simulink model "sim_model_withparasitic_rlload_before"  (R2016a)
settings: Solver=ode4  StartTime=0.0  StopTime=Tfinal  FixedStep=Ts  RelTol=1e-3
values from neighbouring files (symbols this model uses):
  Cdc1 = 5e-6    (= 5e-06)    [sim_parameters.m]    (also in sim_parameters_parallel.m; sim_parameters_rl_load.m)
  delta = acos(Ef/Vt)    [sim_parameters.m]    (also in sim_parameters_parallel.m; sim_parameters_rl_load.m = 0)
  deltad = delta*180/pi    [sim_parameters.m]    (also in sim_parameters_parallel.m; sim_parameters_rl_load.m = 0)
  ESL = 19e-15    (= 1.9e-14)    [sim_parameters.m]    (also in sim_parameters_parallel.m; sim_parameters_rl_load.m = 1e-15)
  ESR = 21.1e-15    (= 2.11e-14)    [sim_parameters.m]    (also in sim_parameters_parallel.m; sim_parameters_rl_load.m = 1e-15)
  LABBot = 10.20e-9    (= 1.02e-08)    [impedance_inductancemodel.m]    (also in sim_parameters_rl_load.m = 1.02e-14)
  LABot = 20.25e-9    (= 2.025e-08)    [impedance_inductancemodel.m]    (also in sim_parameters_rl_load.m = 2.025e-14)
  LABTop = 18.30e-9    (= 1.83e-08)    [impedance_inductancemodel.m]    (also in sim_parameters_rl_load.m = 1.83e-14)
  LATop = 03.40e-9    (= 3.4e-09)    [impedance_inductancemodel.m]    (also in sim_parameters_rl_load.m = 3.4e-15)
  LBBot = 20.38e-9    (= 2.038e-08)    [impedance_inductancemodel.m]    (also in sim_parameters_rl_load.m = 2.038e-14)
  LBCBot = 11.14e-9    (= 1.114e-08)    [impedance_inductancemodel.m]    (also in sim_parameters_rl_load.m = 1.114e-14)
  LBTop = 03.38e-9    (= 3.38e-09)    [impedance_inductancemodel.m]    (also in sim_parameters_rl_load.m = 3.38e-15)
  LCBot = 20.94e-9    (= 2.094e-08)    [impedance_inductancemodel.m]    (also in sim_parameters_rl_load.m = 2.094e-14)
  LCTop = 03.41e-9    (= 3.41e-09)    [impedance_inductancemodel.m]    (also in sim_parameters_rl_load.m = 3.41e-15)
  Lin = 1e-15    [sim_parameters.m]    (also in sim_parameters_parallel.m; sim_parameters_rl_load.m = 1e-06)
  Lload = Xload/(2*pi*fout)    [sim_parameters_rl_load.m]
  ma = Vt*sqrt(3)/(Vdcm*0.612)    [sim_parameters.m]    (also in sim_parameters_parallel.m; sim_parameters_rl_load.m = 0.9)
  maxlim = 340    [sim_parameters.m]    (also in sim_parameters_parallel.m; sim_parameters_rl_load.m)
  minlim = 200    [sim_parameters.m]    (also in sim_parameters_parallel.m; sim_parameters_rl_load.m)
  phase = [0 90 0 90]    [sim_parameters.m]    (also in sim_parameters_parallel.m = [0 0]; sim_parameters_rl_load.m = [0 0])
  RABBot = 10.20e-15    (= 1.02e-14)    [sim_parameters_rl_load.m]
  RABot = 20.25e-15    (= 2.025e-14)    [sim_parameters_rl_load.m]
  RABTop = 18.30e-15    (= 1.83e-14)    [sim_parameters_rl_load.m]
  RATop = 03.40e-15    (= 3.4e-15)    [sim_parameters_rl_load.m]
  RBBot = 20.38e-15    (= 2.038e-14)    [sim_parameters_rl_load.m]
  RBCBot = 11.14e-15    (= 1.114e-14)    [sim_parameters_rl_load.m]
  RBCTop = 21.84e-15    (= 2.184e-14)    [sim_parameters_rl_load.m]
  RBTop = 03.38e-15    (= 3.38e-15)    [sim_parameters_rl_load.m]
  RCBot = 20.94e-15    (= 2.094e-14)    [sim_parameters_rl_load.m]
  RCTop = 03.41e-15    (= 3.41e-15)    [sim_parameters_rl_load.m]
  Rin = 70    [sim_parameters.m]    (also in sim_parameters_parallel.m = 50; sim_parameters_rl_load.m = 200)
  Ripth = 0.3    [sim_parameters.m]    (also in sim_parameters_parallel.m; sim_parameters_rl_load.m = 0.03)
  Rload = Zload*pf    [sim_parameters_rl_load.m]
  Ts = 1e-6    (= 1e-06)    [sim_parameters.m]    (also in sim_parameters_parallel.m = 1e-07; sim_parameters_rl_load.m = 1e-08)
  Vin = Vdc + Rin*(Pout/Vdc)    (= 1751.48148148)    [sim_parameters_rl_load.m]
  wout = 2*pi*fout    (= 314.159265359)    [sim_parameters.m]    (also in sim_parameters_parallel.m; sim_parameters_rl_load.m)
libraries: powerlib x38, powerlib_meascontrol x9, simulink x2
settings Model: SimulationMode=accelerator  Creator=ugurm  LastModifiedBy=mesutto
settings DataIOCC: LimitDataPoints=on  SaveFormat=Array
settings OptimizationCC: EfficientMapNaN2IntZero=off
settings DebuggingCC: UnderspecifiedInitializationDetection=Classic  MergeDetectMultiDrivingBlocksExec=none  SolverPrmCheckMsg=warning  StateNameClashWarn=warning
settings HardwareCC: ProdBitPerPointer=32  ProdLargestAtomicFloat=None  ProdIntDivRoundTo=Undefined  ProdEndianess=Unspecified  ProdWordSize=32  ProdHWDeviceType=32-bit Generic  TargetBitPerPointer=64  TargetLongLongMode=on  TargetIntDivRoundTo=Zero  TargetEndianess=LittleEndian  TargetWordSize=64  TargetHWDeviceType=MATLAB Host  ProdEqTarget=off
settings ModelReferenceCC: PropagateSignalLabelsOutOfModel=off
settings CodeAppCC: MaxIdLength=128
settings GRTTargetCC: GeneratePreprocessorConditionals=Use local settings  CombineOutputUpdateFcns=off  GRTInterface=on
settings ConfigComp: CovModelRefEnable=Off

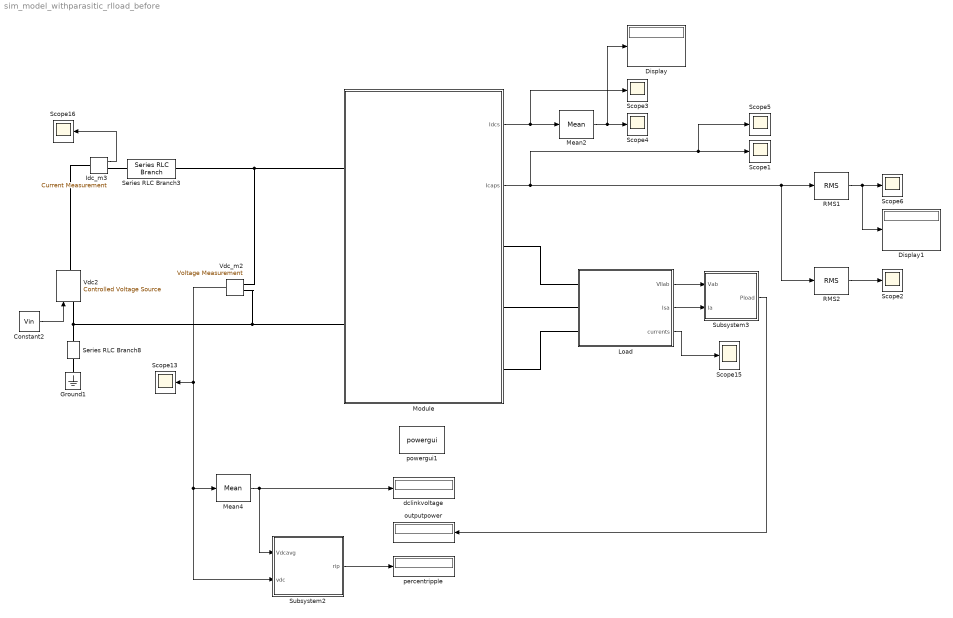
== system sim_model_withparasitic_rlload_before ==
  Constant2 : Constant  Value=Vin
  Display : Display
  Display1 : Display
  Ground1 : powerlib/Elements/Ground  LConnTagsString=a
  Idc_m3 : powerlib/Measurements/Current Measurement  PhasorSimulation=off  OutputType=Complex  PSBequivalent=0
  Load : Subsystem
  Mean2 : powerlib_meascontrol/Measurements/Mean  Freq=fout  Vinit=0  Ts=0
  Mean4 : powerlib_meascontrol/Measurements/Mean  Freq=fout  Vinit=0  Ts=0
  Module : Subsystem
  RMS1 : powerlib_meascontrol/Measurements/RMS  TrueRMS=on  Freq=fout  RMSInit=0  Ts=0
  RMS2 : powerlib_meascontrol/Measurements/RMS  TrueRMS=on  Freq=fsw  RMSInit=0  Ts=0
  Scope{1..6,13,15..16} (9 alike) : Scope
  Series RLC Branch3 : powerlib/Elements/Series RLC Branch  LConnTagsString=__new0  RConnTagsString=__new0  BranchType=R  Resistance=Rin  Inductance=Lin  SetiL0=off  InitialCurrent=0  Capacitance=1e-6  Setx0=off  InitialVoltage=0  Measurements=None
  Series RLC Branch8 : powerlib/Elements/Series RLC Branch  LConnTagsString=__new0  RConnTagsString=__new0  BranchType=R  Resistance=1e12  Inductance=Lload  SetiL0=off  InitialCurrent=0  Capacitance=1e-6  Setx0=off  InitialVoltage=0  Measurements=None
  Subsystem2 : Subsystem
  Subsystem3 : Subsystem
  Vdc2 : powerlib/Electrical Sources/Controlled Voltage Source  Initialize=off  Source_Type=DC  Amplitude=200  Phase=0  Frequency=0  Measurements=None
  Vdc_m2 : powerlib/Measurements/Voltage Measurement  PhasorSimulation=off  OutputType=Complex  PSBequivalent=0
  dclinkvoltage : Display
  outputpower : Display
  percentripple : Display
  powergui1 : powerlib/powergui  Priority=1  SimulationMode=Discrete  SolverType=Tustin  SampleTime=Ts  frequency=60  SPID=off  DisableSnubberDevices=off  DisableRonSwitches=off  DisableVfSwitches=off  SwTol=0  DisplayEquations=off  Interpol=off  ExternalGateDelay=off  methode=off  Ts=0  FunctionMessages=off  echomessages=off  HookPort=off  EnableUseOfTLC=off  x0status=blocks  frequencyindice=0  Pbase=100e6  ErrMax=1e-4  Iterations=50  UnitsV=kV  UnitsW=MW  buscounter=0  RestoreLinks=warning  ResistiveCurrentMeasurement=off  Frange=[0:2:500]  Ylog=off  Xlog=on  ShowGrid=off  save=off  variable=ZData  structure=vdc  ZoomFFT=off  StartTime=0.35  cycles=5  DisplayStyle=4  fundamental=50  FreqAxis=off  MaxFrequency=50000  frequencyindicesteady=1  RmsSteady=1  display=off
  wires:
  Constant2/1 -> Vdc2/1
  Mean4/1 -> Subsystem2/1(Vdcavg), dclinkvoltage/1
  Vdc_m2/1 -> Scope13/1, Subsystem2/2(vdc), Mean4/1
  Idc_m3/1 -> Scope16/1
  Subsystem3/1(Pload) -> outputpower/1
  Load/1(Vllab) -> Subsystem3/1(Vab)
  Load/2(Isa) -> Subsystem3/2(Ia)
  Load/3(currents) -> Scope15/1
  Module/1(Idcs) -> Mean2/1, Scope3/1
  Mean2/1 -> Display/1, Scope4/1
  Module/2(Icaps) -> RMS2/1, RMS1/1, Scope1/1, Scope5/1
  RMS1/1 -> Display1/1, Scope6/1
  Subsystem2/1(rip) -> percentripple/1
  RMS2/1 -> Scope2/1
  connections:
  Series RLC Branch8/RConn1 -- Ground1/LConn1
  Idc_m3/RConn1 -- Series RLC Branch3/LConn1
  Idc_m3/LConn1 -- Vdc2/RConn1
  Vdc_m2/LConn2 -- Module/LConn2 -- Series RLC Branch8/LConn1 -- Vdc2/LConn1
  Vdc_m2/LConn1 -- Series RLC Branch3/RConn1 -- Module/LConn1
  Load/LConn1 -- Module/RConn1
  Load/LConn2 -- Module/RConn2
  Load/LConn3 -- Module/RConn3

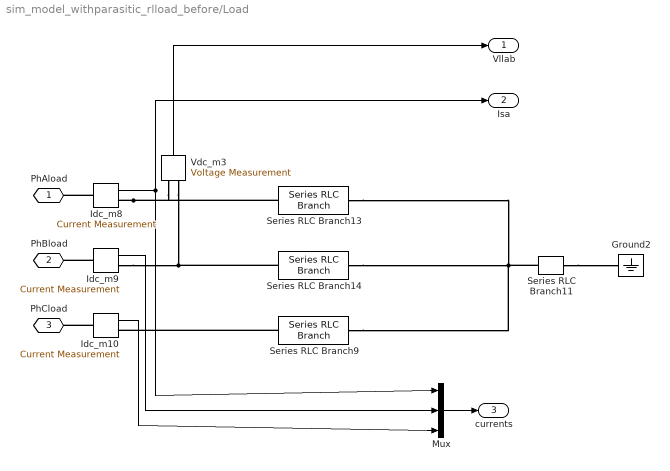
== system sim_model_withparasitic_rlload_before/Load ==
  Ground2 : powerlib/Elements/Ground  LConnTagsString=a
  Idc_m10 : powerlib/Measurements/Current Measurement  PhasorSimulation=off  OutputType=Complex  PSBequivalent=0
  Idc_m8 : powerlib/Measurements/Current Measurement  PhasorSimulation=off  OutputType=Complex  PSBequivalent=0
  Idc_m9 : powerlib/Measurements/Current Measurement  PhasorSimulation=off  OutputType=Complex  PSBequivalent=0
  Mux : Mux  Inputs=3
  Series RLC Branch11 : powerlib/Elements/Series RLC Branch  LConnTagsString=__new0  RConnTagsString=__new0  BranchType=R  Resistance=1e12  Inductance=Lload  SetiL0=off  InitialCurrent=0  Capacitance=1e-6  Setx0=off  InitialVoltage=0  Measurements=None
  Series RLC Branch13 : powerlib/Elements/Series RLC Branch  LConnTagsString=__new0  RConnTagsString=__new0  BranchType=RL  Resistance=Rload  Inductance=Lload  SetiL0=off  InitialCurrent=0  Capacitance=1e-6  Setx0=off  InitialVoltage=0  Measurements=None
  Series RLC Branch14 : powerlib/Elements/Series RLC Branch  LConnTagsString=__new0  RConnTagsString=__new0  BranchType=RL  Resistance=Rload  Inductance=Lload  SetiL0=off  InitialCurrent=0  Capacitance=1e-6  Setx0=off  InitialVoltage=0  Measurements=None
  Series RLC Branch9 : powerlib/Elements/Series RLC Branch  LConnTagsString=__new0  RConnTagsString=__new0  BranchType=RL  Resistance=Rload  Inductance=Lload  SetiL0=off  InitialCurrent=0  Capacitance=1e-6  Setx0=off  InitialVoltage=0  Measurements=None
  Vdc_m3 : powerlib/Measurements/Voltage Measurement  PhasorSimulation=off  OutputType=Complex  PSBequivalent=0
  PhAload : PMIOPort  Port=1  Side=Left
  PhBload : PMIOPort  Port=2  Side=Left
  PhCload : PMIOPort  Port=3  Side=Left
  Vllab : Outport
  Isa : Outport  Port=2
  currents : Outport  Port=3
  wires:
  Vdc_m3/1 -> Vllab/1
  Idc_m9/1 -> Mux/2
  Idc_m10/1 -> Mux/3
  Idc_m8/1 -> Mux/1, Isa/1
  Mux/1 -> currents/1
  connections:
  Idc_m10/LConn1 -- PhCload/RConn1
  Idc_m9/LConn1 -- PhBload/RConn1
  Idc_m8/LConn1 -- PhAload/RConn1
  Series RLC Branch9/LConn1 -- Idc_m10/RConn1
  Vdc_m3/LConn2 -- Idc_m9/RConn1 -- Series RLC Branch14/LConn1
  Series RLC Branch13/RConn1 -- Series RLC Branch9/RConn1 -- Series RLC Branch11/LConn1 -- Series RLC Branch14/RConn1
  Idc_m8/RConn1 -- Vdc_m3/LConn1 -- Series RLC Branch13/LConn1
  Series RLC Branch11/RConn1 -- Ground2/LConn1

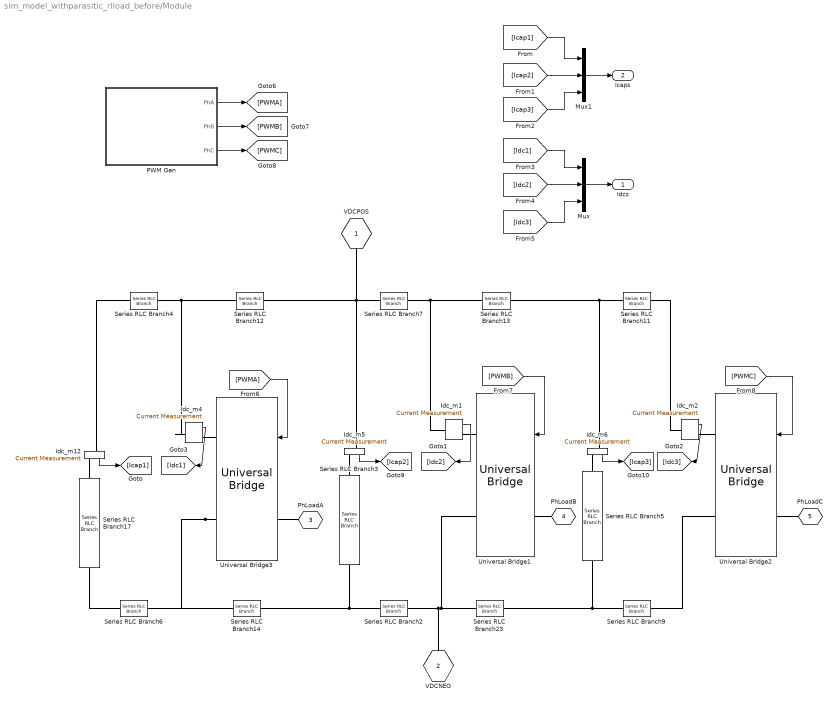
== system sim_model_withparasitic_rlload_before/Module ==
  Idc_m{1..2,4..6,12} (6 alike) : powerlib/Measurements/Current Measurement  PhasorSimulation=off  OutputType=Complex  PSBequivalent=0
  Mux : Mux  Inputs=3
  Mux1 : Mux  Inputs=3
  PWM Gen : Subsystem
  Series RLC Branch11 : powerlib/Elements/Series RLC Branch  LConnTagsString=__new0  RConnTagsString=__new0  BranchType=RL  Resistance=RCTop  Inductance=LCTop  SetiL0=off  InitialCurrent=0  Capacitance=1e-6  Setx0=off  InitialVoltage=0  Measurements=None
  Series RLC Branch12 : powerlib/Elements/Series RLC Branch  LConnTagsString=__new0  RConnTagsString=__new0  BranchType=RL  Resistance=RABTop  Inductance=LABTop  SetiL0=off  InitialCurrent=0  Capacitance=1e-6  Setx0=off  InitialVoltage=0  Measurements=None
  Series RLC Branch13 : powerlib/Elements/Series RLC Branch  LConnTagsString=__new0  RConnTagsString=__new0  BranchType=RL  Resistance=RBCTop  Inductance=RBCTop  SetiL0=off  InitialCurrent=0  Capacitance=1e-6  Setx0=off  InitialVoltage=0  Measurements=None
  Series RLC Branch14 : powerlib/Elements/Series RLC Branch  LConnTagsString=__new0  RConnTagsString=__new0  BranchType=RL  Resistance=RABBot  Inductance=LABBot  SetiL0=off  InitialCurrent=0  Capacitance=1e-6  Setx0=off  InitialVoltage=0  Measurements=None
  Series RLC Branch17 : powerlib/Elements/Series RLC Branch  LConnTagsString=__new0  RConnTagsString=__new0  BranchType=RLC  Resistance=ESR  Inductance=ESL  SetiL0=off  InitialCurrent=0  Capacitance=Cdc1  Setx0=off  InitialVoltage=0  Measurements=None
  Series RLC Branch2 : powerlib/Elements/Series RLC Branch  LConnTagsString=__new0  RConnTagsString=__new0  BranchType=RL  Resistance=RBBot  Inductance=LBBot  SetiL0=off  InitialCurrent=0  Capacitance=1e-6  Setx0=off  InitialVoltage=0  Measurements=None
  Series RLC Branch23 : powerlib/Elements/Series RLC Branch  LConnTagsString=__new0  RConnTagsString=__new0  BranchType=RL  Resistance=RBCBot  Inductance=LBCBot  SetiL0=off  InitialCurrent=0  Capacitance=1e-6  Setx0=off  InitialVoltage=0  Measurements=None
  Series RLC Branch3 : powerlib/Elements/Series RLC Branch  LConnTagsString=__new0  RConnTagsString=__new0  BranchType=RLC  Resistance=ESR  Inductance=ESL  SetiL0=off  InitialCurrent=0  Capacitance=Cdc1  Setx0=off  InitialVoltage=0  Measurements=None
  Series RLC Branch4 : powerlib/Elements/Series RLC Branch  LConnTagsString=__new0  RConnTagsString=__new0  BranchType=RL  Resistance=RATop  Inductance=LATop  SetiL0=off  InitialCurrent=0  Capacitance=1e-6  Setx0=off  InitialVoltage=0  Measurements=None
  Series RLC Branch5 : powerlib/Elements/Series RLC Branch  LConnTagsString=__new0  RConnTagsString=__new0  BranchType=RLC  Resistance=ESR  Inductance=ESL  SetiL0=off  InitialCurrent=0  Capacitance=Cdc1  Setx0=off  InitialVoltage=0  Measurements=None
  Series RLC Branch6 : powerlib/Elements/Series RLC Branch  LConnTagsString=__new0  RConnTagsString=__new0  BranchType=RL  Resistance=LABot  Inductance=RABot  SetiL0=off  InitialCurrent=0  Capacitance=1e-6  Setx0=off  InitialVoltage=0  Measurements=None
  Series RLC Branch7 : powerlib/Elements/Series RLC Branch  LConnTagsString=__new0  RConnTagsString=__new0  BranchType=RL  Resistance=RBTop  Inductance=LBTop  SetiL0=off  InitialCurrent=0  Capacitance=1e-6  Setx0=off  InitialVoltage=0  Measurements=None
  Series RLC Branch9 : powerlib/Elements/Series RLC Branch  LConnTagsString=__new0  RConnTagsString=__new0  BranchType=RL  Resistance=RCBot  Inductance=LCBot  SetiL0=off  InitialCurrent=0  Capacitance=1e-6  Setx0=off  InitialVoltage=0  Measurements=None
  Universal Bridge1 : powerlib/Power Electronics/Universal Bridge  Arms=1  SnubberResistance=1e5  SnubberCapacitance=inf  Device=IGBT / Diodes  Ron=1e-6  Lon=0  ForwardVoltages="[  0  0  ]"  ForwardVoltage=0  GTOparameters=[ 10e-6 , 20e-6 ]  IGBTparameters=[ 1e-6 , 2e-6 ]  Measurements=None  Measurements_2=None  converterType=Rectifier
  Universal Bridge2 : powerlib/Power Electronics/Universal Bridge  Arms=1  SnubberResistance=1e5  SnubberCapacitance=inf  Device=IGBT / Diodes  Ron=1e-6  Lon=0  ForwardVoltages="[  0  0  ]"  ForwardVoltage=0  GTOparameters=[ 10e-6 , 20e-6 ]  IGBTparameters=[ 1e-6 , 2e-6 ]  Measurements=None  Measurements_2=None  converterType=Rectifier
  Universal Bridge3 : powerlib/Power Electronics/Universal Bridge  Arms=1  SnubberResistance=1e5  SnubberCapacitance=inf  Device=IGBT / Diodes  Ron=1e-6  Lon=0  ForwardVoltages="[  0  0  ]"  ForwardVoltage=0  GTOparameters=[ 10e-6 , 20e-6 ]  IGBTparameters=[ 1e-6 , 2e-6 ]  Measurements=None  Measurements_2=None  converterType=Rectifier
  VDCPOS : PMIOPort  Port=1  Side=Left
  VDCNEG : PMIOPort  Port=2  Side=Left
  PhLoadA : PMIOPort  Port=3  Side=Right
  PhLoadB : PMIOPort  Port=4  Side=Right
  PhLoadC : PMIOPort  Port=5  Side=Right
  Idcs : Outport
  Icaps : Outport  Port=2
  wires:
  Idc_m5/1 -> [Icap2]
  Idc_m12/1 -> [Icap1]
  [PWMA] -> Universal Bridge3/1
  [PWMC] -> Universal Bridge2/1
  [PWMB] -> Universal Bridge1/1
  Idc_m6/1 -> [Icap3]
  Idc_m4/1 -> [Idc1]
  Idc_m1/1 -> [Idc2]
  Idc_m2/1 -> [Idc3]
  PWM Gen/1(PhA) -> [PWMA]
  PWM Gen/2(PhB) -> [PWMB]
  PWM Gen/3(PhC) -> [PWMC]
  Mux/1 -> Idcs/1
  Mux1/1 -> Icaps/1
  [Icap2] -> Mux1/2
  [Icap1] -> Mux1/1
  [Icap3] -> Mux1/3
  [Idc2] -> Mux/2
  [Idc1] -> Mux/1
  [Idc3] -> Mux/3
  connections:
  Idc_m12/LConn1 -- Series RLC Branch4/RConn1
  Idc_m6/LConn1 -- Series RLC Branch13/LConn1 -- Series RLC Branch11/RConn1
  Idc_m5/LConn1 -- VDCPOS/RConn1 -- Series RLC Branch7/RConn1 -- Series RLC Branch12/LConn1
  Series RLC Branch13/RConn1 -- Idc_m1/LConn1 -- Series RLC Branch7/LConn1
  Series RLC Branch3/LConn1 -- Idc_m5/RConn1
  Series RLC Branch4/LConn1 -- Idc_m4/LConn1 -- Series RLC Branch12/RConn1
  PhLoadB/RConn1 -- Universal Bridge1/LConn1
  Idc_m12/RConn1 -- Series RLC Branch17/LConn1
  PhLoadC/RConn1 -- Universal Bridge2/LConn1
  Series RLC Branch5/LConn1 -- Idc_m6/RConn1
  Universal Bridge2/RConn2 -- Series RLC Branch9/LConn1
  PhLoadA/RConn1 -- Universal Bridge3/LConn1
  Series RLC Branch6/RConn1 -- Series RLC Branch17/RConn1
  Universal Bridge3/RConn2 -- Series RLC Branch6/LConn1 -- Series RLC Branch14/RConn1
  Series RLC Branch14/LConn1 -- Series RLC Branch3/RConn1 -- Series RLC Branch2/RConn1
  Series RLC Branch2/LConn1 -- VDCNEG/RConn1 -- Series RLC Branch23/RConn1 -- Universal Bridge1/RConn2
  Series RLC Branch23/LConn1 -- Series RLC Branch5/RConn1 -- Series RLC Branch9/RConn1
  Idc_m4/RConn1 -- Universal Bridge3/RConn1
  Universal Bridge1/RConn1 -- Idc_m1/RConn1
  Universal Bridge2/RConn1 -- Idc_m2/RConn1
  Series RLC Branch11/LConn1 -- Idc_m2/LConn1

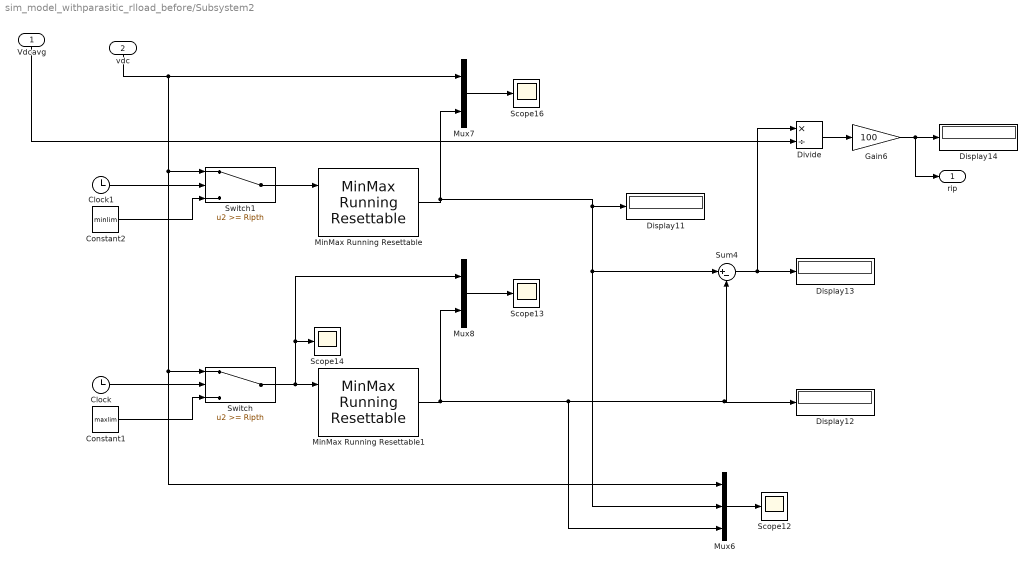
== system sim_model_withparasitic_rlload_before/Subsystem2 ==
  Vdcavg : Inport
  vdc : Inport  Port=2
  Clock : Clock
  Clock1 : Clock
  Constant1 : Constant  Value=maxlim  SampleTime=Ts
  Constant2 : Constant  Value=minlim  SampleTime=Ts
  Display{11..14} (4 alike) : Display
  Divide : Product  Inputs=*/
  Gain6 : Gain  Gain=100
  MinMax Running Resettable : simulink/Math Operations/MinMax Running Resettable  Function=max  vinit=0.0
  MinMax Running Resettable1 : simulink/Math Operations/MinMax Running Resettable  Function=min  vinit=700
  Mux6 : Mux  Inputs=3
  Mux7 : Mux  Inputs=2
  Mux8 : Mux  Inputs=2
  Scope{12..14,16} (4 alike) : Scope
  Sum4 : Sum  Inputs=|+-
  Switch : Switch  Threshold=Ripth
  Switch1 : Switch  Threshold=Ripth
  rip : Outport
  wires:
  MinMax Running Resettable/1 -> Display11/1, Mux6/2, Sum4/1, Mux7/2
  Clock/1 -> Switch/2
  Mux8/1 -> Scope13/1
  Gain6/1 -> rip/1, Display14/1
  Constant1/1 -> Switch/3
  MinMax Running Resettable1/1 -> Mux6/3, Display12/1, Sum4/2, Mux8/2
  Mux7/1 -> Scope16/1
  Switch/1 -> Mux8/1, Scope14/1, MinMax Running Resettable1/1
  Sum4/1 -> Divide/1, Display13/1
  Divide/1 -> Gain6/1
  Mux6/1 -> Scope12/1
  Vdcavg/1 -> Divide/2
  vdc/1 -> Mux7/1, Switch1/1, Mux6/1, Switch/1
  Switch1/1 -> MinMax Running Resettable/1
  Clock1/1 -> Switch1/2
  Constant2/1 -> Switch1/3

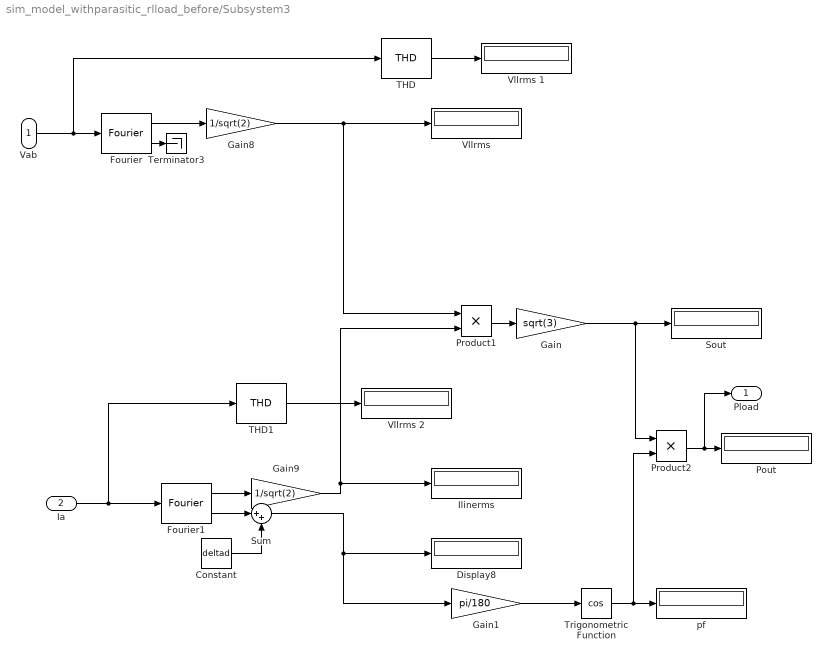
== system sim_model_withparasitic_rlload_before/Subsystem3 ==
  Vab : Inport
  Ia : Inport  Port=2
  Constant : Constant  Value=deltad
  Display8 : Display
  Fourier : powerlib_meascontrol/Measurements/Fourier  Freq=fout  n=1  InInit=[0, 0]  Ts=Ts
  Fourier1 : powerlib_meascontrol/Measurements/Fourier  Freq=fout  n=1  InInit=[0, 0]  Ts=Ts
  Gain : Gain  Gain=sqrt(3)
  Gain1 : Gain  Gain=pi/180
  Gain8 : Gain  Gain=1/sqrt(2)
  Gain9 : Gain  Gain=1/sqrt(2)
  "Ilinerms " : Display
  Pout : Display
  Product1 : Product
  Product2 : Product
  Sout : Display
      settings: Format=short_e
  Sum : Sum  Inputs=|++
  THD : powerlib_meascontrol/Measurements/THD  Freq=fout  Ts=0
  THD1 : powerlib_meascontrol/Measurements/THD  Freq=fout  Ts=0
  Terminator3 : Terminator
  Trigonometric Function : Trigonometry  Operator=cos
  "Vllrms " : Display
  Vllrms 1 : Display
  Vllrms 2 : Display
  pf : Display
  Pload : Outport
  wires:
  Gain8/1 -> Product1/1, "Vllrms "/1
  Gain9/1 -> "Ilinerms "/1, Product1/2
  Ia/1 -> THD1/1, Fourier1/1
  Fourier1/1 -> Gain9/1
  Vab/1 -> THD/1, Fourier/1
  Fourier/1 -> Gain8/1
  Product1/1 -> Gain/1
  Gain/1 -> Product2/1, Sout/1
  Sum/1 -> Gain1/1, Display8/1
  Trigonometric Function/1 -> Product2/2, pf/1
  Gain1/1 -> Trigonometric Function/1
  Product2/1 -> Pload/1, Pout/1
  Fourier/2 -> Terminator3/1
  THD/1 -> Vllrms 1/1
  THD1/1 -> Vllrms 2/1
  Fourier1/2 -> Sum/1
  Constant/1 -> Sum/2

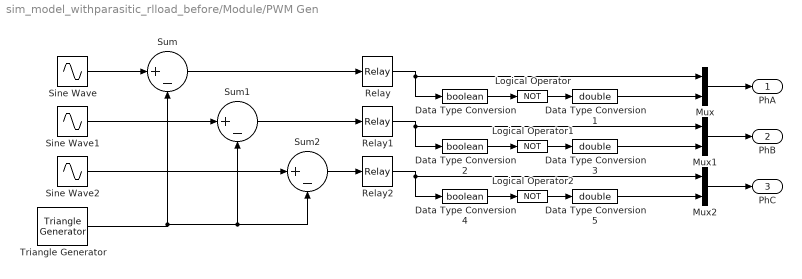
== system sim_model_withparasitic_rlload_before/Module/PWM Gen ==
  Data Type Conversion : DataTypeConversion  OutDataTypeStr=boolean
  Data Type Conversion1 : DataTypeConversion  OutDataTypeStr=double
  Data Type Conversion2 : DataTypeConversion  OutDataTypeStr=boolean
  Data Type Conversion3 : DataTypeConversion  OutDataTypeStr=double
  Data Type Conversion4 : DataTypeConversion  OutDataTypeStr=boolean
  Data Type Conversion5 : DataTypeConversion  OutDataTypeStr=double
  Logical Operator : Logic  Operator=NOT  AllPortsSameDT=off  OutDataTypeStr=boolean
  Logical Operator1 : Logic  Operator=NOT  AllPortsSameDT=off  OutDataTypeStr=boolean
  Logical Operator2 : Logic  Operator=NOT  AllPortsSameDT=off  OutDataTypeStr=boolean
  Mux : Mux  Inputs=2
  Mux1 : Mux  Inputs=2
  Mux2 : Mux  Inputs=2
  Relay : Relay
  Relay1 : Relay
  Relay2 : Relay
  Sine Wave : Sin  Amplitude=ma  Frequency=wout  Phase=delta  SampleTime=0
  Sine Wave1 : Sin  Amplitude=ma  Frequency=wout  Phase=-2*pi/3+delta  SampleTime=0
  Sine Wave2 : Sin  Amplitude=ma  Frequency=wout  Phase=2*pi/3+delta  SampleTime=0
  Sum : Sum  Inputs=|+-
  Sum1 : Sum  Inputs=|+-
  Sum2 : Sum  Inputs=|+-
  Triangle Generator : powerlib_meascontrol/Pulse & Signal Generators/Triangle Generator  Freq=fsw  Phase=phase(1)  Ts=Ts
  PhA : Outport
  PhB : Outport  Port=2
  PhC : Outport  Port=3
  wires:
  Sine Wave1/1 -> Sum1/1
  Sine Wave2/1 -> Sum2/1
  Logical Operator/1 -> Data Type Conversion1/1
  Data Type Conversion2/1 -> Logical Operator1/1
  Relay1/1 -> Data Type Conversion2/1, Mux1/1
  Logical Operator1/1 -> Data Type Conversion3/1
  Sum2/1 -> Relay2/1
  Data Type Conversion4/1 -> Logical Operator2/1
  Logical Operator2/1 -> Data Type Conversion5/1
  Sum/1 -> Relay/1
  Data Type Conversion/1 -> Logical Operator/1
  Relay/1 -> Mux/1, Data Type Conversion/1
  Triangle Generator/1 -> Sum1/2, Sum2/2, Sum/2
  Sum1/1 -> Relay1/1
  Data Type Conversion1/1 -> Mux/2
  Relay2/1 -> Data Type Conversion4/1, Mux2/1
  Sine Wave/1 -> Sum/1
  Mux/1 -> PhA/1
  Mux1/1 -> PhB/1
  Data Type Conversion3/1 -> Mux1/2
  Mux2/1 -> PhC/1
  Data Type Conversion5/1 -> Mux2/2
